simulink model "Heating_system"  (R2021a)
settings: Solver=VariableStepAuto  StartTime=0.0  StopTime=10.0  RelTol=1e-3
model workspace (MAT data in the model file):
  H = Simulink.Bus
  H.Alignment = -1
  H.PreserveElementDimensions = 0
  H.DataScope = 'Auto'
settings Model: OrderedModelArguments=off  Creator=smrh1  LastModifiedBy=smrh1

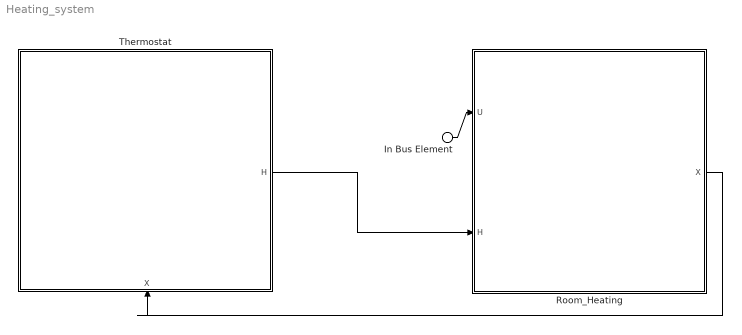
== system Heating_system ==
  In Bus Element : Inport  PortName=U
  Room_Heating : Subsystem
      settings: PortSchema="{\"entries\":[{\"content\":{\"headerSize\":26,\"margin\":15,\"minimumSpacing\":25,\"sides\":[{\"content\":{\"connectorIds\":[\"In1\",\"In2\"]},\"type\":\"ConnectorPlacement.EquallySpacedRectSide\",\"uuid\":\"3399fd0f-e173-41a6-b187-8436c8bfa551\"},{\"content\":{\"connectorIds\":[\"Out1\"],\"side\":\"RIGHT\"},\"type\":\"ConnectorPlacement.EquallySpacedRectSide\",\"uuid\":\"ade3010a-e700-4d19-9692-9b4fbd9f77bd\"},{\"content\":{\"connectorIds\":[],\"side\":\"TOP\"},\"type\":\"ConnectorPlacement.EquallySpacedRectSide\",\"uuid\":\"996f7f95-9ab9-4e94-926a-d72fb20bb1ec\"}]},\"type\":\"ConnectorPlacement.EquallySpacedConnector\",\"uuid\":\"0c58a4e7-12d7-4b31-b33f-6c78252624a7\"}],\"packageUris\":[\"http://schema.mathworks.com/mf0/Connector/R2020b\"],\"version\":\"1.0\"}"
  Thermostat : Subsystem
      settings: PortSchema="{\"entries\":[{\"content\":{\"headerSize\":26,\"margin\":15,\"minimumSpacing\":25,\"sides\":[{\"content\":{\"connectorIds\":[]},\"type\":\"ConnectorPlacement.EquallySpacedRectSide\",\"uuid\":\"3399fd0f-e173-41a6-b187-8436c8bfa551\"},{\"content\":{\"connectorIds\":[\"Out1\"],\"side\":\"RIGHT\"},\"type\":\"ConnectorPlacement.EquallySpacedRectSide\",\"uuid\":\"ade3010a-e700-4d19-9692-9b4fbd9f77bd\"},{\"content\":{\"connectorIds\":[],\"side\":\"TOP\"},\"type\":\"ConnectorPlacement.EquallySpacedRectSide\",\"uuid\":\"996f7f95-9ab9-4e94-926a-d72fb20bb1ec\"},{\"content\":{\"connectorIds\":[\"In1\"],\"side\":\"BOTTOM\"},\"type\":\"ConnectorPlacement.EquallySpacedRectSide\",\"uuid\":\"850434b0-8785-4975-a631-b4ec0ca1fe29\"}]},\"type\":\"ConnectorPlacement.EquallySpacedConnector\",\"uuid\":\"0c58a4e7-12d7-4b31-b33f-6c78252624a7\"}],\"packageUris\":[\"http://schema.mathworks.com/mf0/Connector/R2020b\"],\"version\":\"1.0\"}"
  wires:
  Thermostat/1(H) -> Room_Heating/2(H)
  In Bus Element/1 -> Room_Heating/1(U)
  Room_Heating/1(X) -> Thermostat/1(X)

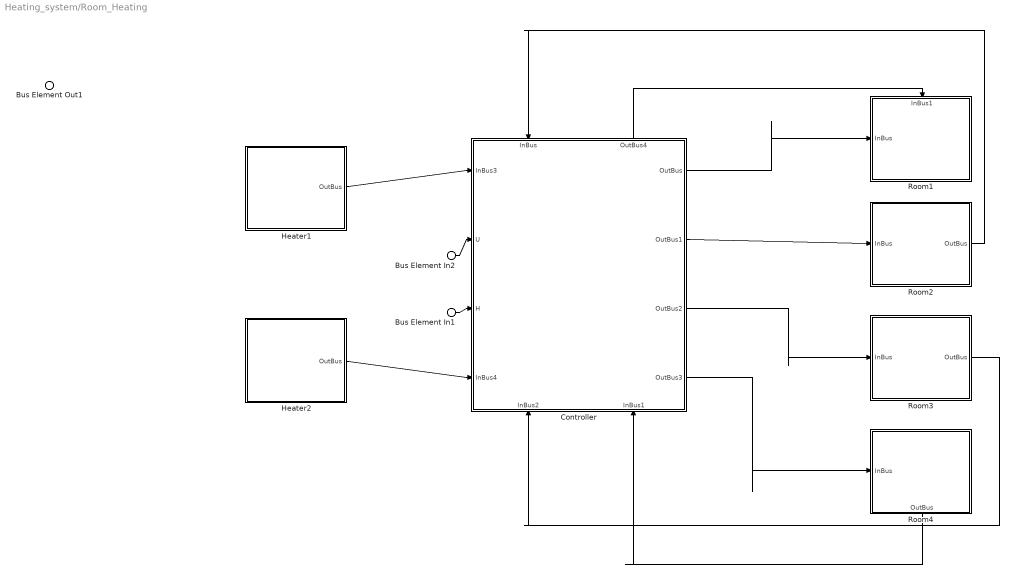
== system Heating_system/Room_Heating ==
  Bus Element In2 : Inport  PortName=U
  Bus Element In1 : Inport  Port=2  PortName=H
  Controller : Subsystem
      settings: PortSchema="{\"entries\":[{\"content\":{\"headerSize\":26,\"margin\":15,\"minimumSpacing\":25,\"sides\":[{\"content\":{\"connectorIds\":[\"In1\",\"In6\",\"In7\",\"In4\"]},\"type\":\"ConnectorPlacement.EquallySpacedRectSide\",\"uuid\":\"3399fd0f-e173-41a6-b187-8436c8bfa551\"},{\"content\":{\"connectorIds\":[\"Out2\",\"Out3\",\"Out4\",\"Out5\"],\"side\":\"RIGHT\"},\"type\":\"ConnectorPlacement.EquallySpacedRectSide\",\"uuid\":\"ade3010a-e700-4d19-9692-9b4fbd9f77bd\"},{\"content\":{\"connectorIds\":[\"In5\",\"Out1\"],\"side\":\"TOP\"},\"type\":\"ConnectorPlacement.EquallySpacedRectSide\",\"uuid\":\"996f7f95-9ab9-4e94-926a-d72fb20bb1ec\"},{\"content\":{\"connectorIds\":[\"In2\",\"In3\"],\"side\":\"BOTTOM\"},\"type\":\"ConnectorPlacement.EquallySpacedRectSide\",\"uuid\":\"d0b71253-16d9-4f1a-b9f2-f0c88116a428\"}]},\"type\":\"ConnectorPlacement.EquallySpacedConnector\",\"uuid\":\"0c58a4e7-12d7-4b31-b33f-6c78252624a7\"}],\"packageUris\":[\"http://schema.mathworks.com/mf0/Connector/R2020b\"],\"version\":\"1.0\"}"
  Heater1 : Subsystem
      settings: PortSchema="{\"entries\":[{\"content\":{\"headerSize\":26,\"margin\":15,\"minimumSpacing\":25,\"sides\":[{\"content\":{\"connectorIds\":[]},\"type\":\"ConnectorPlacement.EquallySpacedRectSide\",\"uuid\":\"3399fd0f-e173-41a6-b187-8436c8bfa551\"},{\"content\":{\"connectorIds\":[\"Out1\"],\"side\":\"RIGHT\"},\"type\":\"ConnectorPlacement.EquallySpacedRectSide\",\"uuid\":\"ade3010a-e700-4d19-9692-9b4fbd9f77bd\"},{\"content\":{\"connectorIds\":[],\"side\":\"TOP\"},\"type\":\"ConnectorPlacement.EquallySpacedRectSide\",\"uuid\":\"996f7f95-9ab9-4e94-926a-d72fb20bb1ec\"}]},\"type\":\"ConnectorPlacement.EquallySpacedConnector\",\"uuid\":\"0c58a4e7-12d7-4b31-b33f-6c78252624a7\"}],\"packageUris\":[\"http://schema.mathworks.com/mf0/Connector/R2020b\"],\"version\":\"1.0\"}"
  Heater2 : Subsystem
      settings: PortSchema="{\"entries\":[{\"content\":{\"headerSize\":26,\"margin\":15,\"minimumSpacing\":25,\"sides\":[{\"content\":{\"connectorIds\":[]},\"type\":\"ConnectorPlacement.EquallySpacedRectSide\",\"uuid\":\"3399fd0f-e173-41a6-b187-8436c8bfa551\"},{\"content\":{\"connectorIds\":[\"Out1\"],\"side\":\"RIGHT\"},\"type\":\"ConnectorPlacement.EquallySpacedRectSide\",\"uuid\":\"ade3010a-e700-4d19-9692-9b4fbd9f77bd\"},{\"content\":{\"connectorIds\":[],\"side\":\"TOP\"},\"type\":\"ConnectorPlacement.EquallySpacedRectSide\",\"uuid\":\"996f7f95-9ab9-4e94-926a-d72fb20bb1ec\"}]},\"type\":\"ConnectorPlacement.EquallySpacedConnector\",\"uuid\":\"0c58a4e7-12d7-4b31-b33f-6c78252624a7\"}],\"packageUris\":[\"http://schema.mathworks.com/mf0/Connector/R2020b\"],\"version\":\"1.0\"}"
  Room1 : Subsystem
      settings: PortSchema="{\"entries\":[{\"content\":{\"headerSize\":26,\"margin\":15,\"minimumSpacing\":25,\"sides\":[{\"content\":{\"connectorIds\":[\"In2\"]},\"type\":\"ConnectorPlacement.EquallySpacedRectSide\",\"uuid\":\"3399fd0f-e173-41a6-b187-8436c8bfa551\"},{\"content\":{\"connectorIds\":[],\"side\":\"RIGHT\"},\"type\":\"ConnectorPlacement.EquallySpacedRectSide\",\"uuid\":\"ade3010a-e700-4d19-9692-9b4fbd9f77bd\"},{\"content\":{\"connectorIds\":[\"In1\"],\"side\":\"TOP\"},\"type\":\"ConnectorPlacement.EquallySpacedRectSide\",\"uuid\":\"996f7f95-9ab9-4e94-926a-d72fb20bb1ec\"}]},\"type\":\"ConnectorPlacement.EquallySpacedConnector\",\"uuid\":\"0c58a4e7-12d7-4b31-b33f-6c78252624a7\"}],\"packageUris\":[\"http://schema.mathworks.com/mf0/Connector/R2020b\"],\"version\":\"1.0\"}"
  Room2 : Subsystem
      settings: PortSchema="{\"entries\":[{\"content\":{\"headerSize\":26,\"margin\":15,\"minimumSpacing\":25,\"sides\":[{\"content\":{\"connectorIds\":[\"In1\"]},\"type\":\"ConnectorPlacement.EquallySpacedRectSide\",\"uuid\":\"3399fd0f-e173-41a6-b187-8436c8bfa551\"},{\"content\":{\"connectorIds\":[\"Out1\"],\"side\":\"RIGHT\"},\"type\":\"ConnectorPlacement.EquallySpacedRectSide\",\"uuid\":\"ade3010a-e700-4d19-9692-9b4fbd9f77bd\"},{\"content\":{\"connectorIds\":[],\"side\":\"TOP\"},\"type\":\"ConnectorPlacement.EquallySpacedRectSide\",\"uuid\":\"996f7f95-9ab9-4e94-926a-d72fb20bb1ec\"}]},\"type\":\"ConnectorPlacement.EquallySpacedConnector\",\"uuid\":\"0c58a4e7-12d7-4b31-b33f-6c78252624a7\"}],\"packageUris\":[\"http://schema.mathworks.com/mf0/Connector/R2020b\"],\"version\":\"1.0\"}"
  Room3 : Subsystem
      settings: PortSchema="{\"entries\":[{\"content\":{\"headerSize\":26,\"margin\":15,\"minimumSpacing\":25,\"sides\":[{\"content\":{\"connectorIds\":[\"In1\"]},\"type\":\"ConnectorPlacement.EquallySpacedRectSide\",\"uuid\":\"3399fd0f-e173-41a6-b187-8436c8bfa551\"},{\"content\":{\"connectorIds\":[\"Out1\"],\"side\":\"RIGHT\"},\"type\":\"ConnectorPlacement.EquallySpacedRectSide\",\"uuid\":\"ade3010a-e700-4d19-9692-9b4fbd9f77bd\"},{\"content\":{\"connectorIds\":[],\"side\":\"TOP\"},\"type\":\"ConnectorPlacement.EquallySpacedRectSide\",\"uuid\":\"996f7f95-9ab9-4e94-926a-d72fb20bb1ec\"}]},\"type\":\"ConnectorPlacement.EquallySpacedConnector\",\"uuid\":\"0c58a4e7-12d7-4b31-b33f-6c78252624a7\"}],\"packageUris\":[\"http://schema.mathworks.com/mf0/Connector/R2020b\"],\"version\":\"1.0\"}"
  Room4 : Subsystem
      settings: PortSchema="{\"entries\":[{\"content\":{\"headerSize\":26,\"margin\":15,\"minimumSpacing\":25,\"sides\":[{\"content\":{\"connectorIds\":[\"In1\"]},\"type\":\"ConnectorPlacement.EquallySpacedRectSide\",\"uuid\":\"3399fd0f-e173-41a6-b187-8436c8bfa551\"},{\"content\":{\"connectorIds\":[],\"side\":\"RIGHT\"},\"type\":\"ConnectorPlacement.EquallySpacedRectSide\",\"uuid\":\"ade3010a-e700-4d19-9692-9b4fbd9f77bd\"},{\"content\":{\"connectorIds\":[],\"side\":\"TOP\"},\"type\":\"ConnectorPlacement.EquallySpacedRectSide\",\"uuid\":\"996f7f95-9ab9-4e94-926a-d72fb20bb1ec\"},{\"content\":{\"connectorIds\":[\"Out1\"],\"side\":\"BOTTOM\"},\"type\":\"ConnectorPlacement.EquallySpacedRectSide\",\"uuid\":\"5b6f9b21-bc12-41f2-b941-cb072175fade\"}]},\"type\":\"ConnectorPlacement.EquallySpacedConnector\",\"uuid\":\"0c58a4e7-12d7-4b31-b33f-6c78252624a7\"}],\"packageUris\":[\"http://schema.mathworks.com/mf0/Connector/R2020b\"],\"version\":\"1.0\"}"
  Bus Element Out1 : Outport  PortName=X
  wires:
  Bus Element In1/1 -> Controller/7(H)
  Bus Element In2/1 -> Controller/6(U)
  Controller/2(OutBus) -> Room1/2(InBus)
  Controller/3(OutBus1) -> Room2/1(InBus)
  Controller/4(OutBus2) -> Room3/1(InBus)
  Controller/5(OutBus3) -> Room4/1(InBus)
  Controller/1(OutBus4) -> Room1/1(InBus1)
  Room2/1(OutBus) -> Controller/5(InBus)
  Room4/1(OutBus) -> Controller/3(InBus1)
  Room3/1(OutBus) -> Controller/2(InBus2)
  Heater1/1(OutBus) -> Controller/1(InBus3)
  Heater2/1(OutBus) -> Controller/4(InBus4)

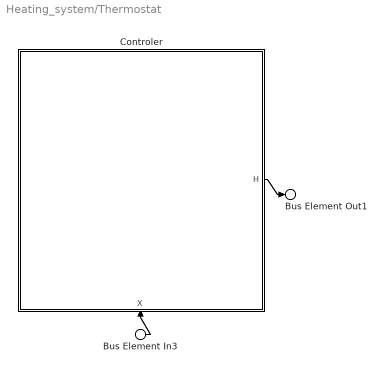
== system Heating_system/Thermostat ==
  Bus Element In3 : Inport  PortName=X
  Controler : Subsystem
      settings: PortSchema="{\"entries\":[{\"content\":{\"headerSize\":26,\"margin\":15,\"minimumSpacing\":25,\"sides\":[{\"content\":{\"connectorIds\":[]},\"type\":\"ConnectorPlacement.EquallySpacedRectSide\",\"uuid\":\"3399fd0f-e173-41a6-b187-8436c8bfa551\"},{\"content\":{\"connectorIds\":[\"Out1\"],\"side\":\"RIGHT\"},\"type\":\"ConnectorPlacement.EquallySpacedRectSide\",\"uuid\":\"ade3010a-e700-4d19-9692-9b4fbd9f77bd\"},{\"content\":{\"connectorIds\":[],\"side\":\"TOP\"},\"type\":\"ConnectorPlacement.EquallySpacedRectSide\",\"uuid\":\"996f7f95-9ab9-4e94-926a-d72fb20bb1ec\"},{\"content\":{\"connectorIds\":[\"In1\"],\"side\":\"BOTTOM\"},\"type\":\"ConnectorPlacement.EquallySpacedRectSide\",\"uuid\":\"af2d879e-2584-461c-b0c1-874abed785b7\"}]},\"type\":\"ConnectorPlacement.EquallySpacedConnector\",\"uuid\":\"0c58a4e7-12d7-4b31-b33f-6c78252624a7\"}],\"packageUris\":[\"http://schema.mathworks.com/mf0/Connector/R2020b\"],\"version\":\"1.0\"}"
  Bus Element Out1 : Outport  PortName=H
  wires:
  Controler/1(H) -> Bus Element Out1/1
  Bus Element In3/1 -> Controler/1(X)

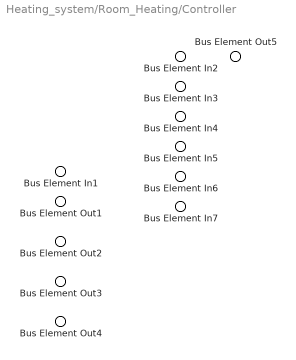
== system Heating_system/Room_Heating/Controller ==
  Bus Element In6 : Inport  PortName=InBus3
  Bus Element In5 : Inport  Port=2  PortName=InBus2
  Bus Element In4 : Inport  Port=3  PortName=InBus1
  Bus Element In7 : Inport  Port=4  PortName=InBus4
  Bus Element In3 : Inport  Port=5  PortName=InBus
  Bus Element In2 : Inport  Port=6  PortName=U
  Bus Element In1 : Inport  Port=7  PortName=H
  Bus Element Out5 : Outport  PortName=OutBus4
  Bus Element Out1 : Outport  Port=2  PortName=OutBus
  Bus Element Out2 : Outport  Port=3  PortName=OutBus1
  Bus Element Out3 : Outport  Port=4  PortName=OutBus2
  Bus Element Out4 : Outport  Port=5  PortName=OutBus3

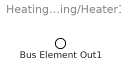
== system Heating_system/Room_Heating/Heater1 ==
  Bus Element Out1 : Outport  PortName=OutBus

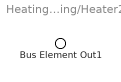
== system Heating_system/Room_Heating/Heater2 ==
  Bus Element Out1 : Outport  PortName=OutBus

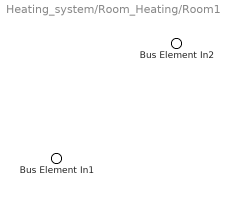
== system Heating_system/Room_Heating/Room1 ==
  Bus Element In2 : Inport  PortName=InBus1
  Bus Element In1 : Inport  Port=2  PortName=InBus

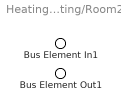
== system Heating_system/Room_Heating/Room2 ==
  Bus Element In1 : Inport  PortName=InBus
  Bus Element Out1 : Outport  PortName=OutBus

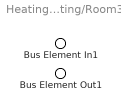
== system Heating_system/Room_Heating/Room3 ==
  Bus Element In1 : Inport  PortName=InBus
  Bus Element Out1 : Outport  PortName=OutBus

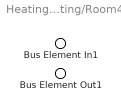
== system Heating_system/Room_Heating/Room4 ==
  Bus Element In1 : Inport  PortName=InBus
  Bus Element Out1 : Outport  PortName=OutBus

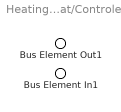
== system Heating_system/Thermostat/Controler ==
  Bus Element In1 : Inport  PortName=X
  Bus Element Out1 : Outport  PortName=H
